simulink model "serial_spi__MAX11300"  (R2016b)
settings: Solver=FixedStepDiscrete  StartTime=0.0  StopTime=50  FixedStep=1e-3  RelTol=1e-3
undefined symbols (not defined in the file or in its folder): Ended, Single
libraries: mbed_spi_max11300 x8, mbed_lib x4
settings Model: Creator=oh  LastModifiedBy=oh
settings DataIOCC: LimitDataPoints=on  SaveFormat=Array
settings OptimizationCC: LifeSpan=1
settings DebuggingCC: SFUnexpectedBacktrackingDiag=warning  SFNoUnconditionalDefaultTransitionDiag=warning  SFExecutionAtInitializationDiag=none
settings HardwareCC: ProdBitPerPointer=32  ProdBitPerSizeT=32  ProdBitPerPtrDiffT=32  ProdLargestAtomicInteger=Long  ProdLargestAtomicFloat=Double  ProdIntDivRoundTo=Undefined  ProdWordSize=32  ProdHWDeviceType=ARM Compatible->ARM Cortex
settings ModelReferenceCC: PropagateSignalLabelsOutOfModel=off
settings RTWCC: SystemTargetFile=mbed.tlc  TemplateMakefile=mbed.tmf  Description=Mbed Target (Embedded Target)  TargetLang=C++
settings CodeAppCC: IgnoreCustomStorageClasses=off
settings STFCustomTargetCC: TargetLibSuffix=.a  GenerateSampleERTMain=on  CombineOutputUpdateFcns=on  ERTCustomFileBanners=on  SupportContinuousTime=off  SupportNonInlinedSFcns=off  RemoveResetFunc=on  MATLABClassNameForMDSCustomization=Simulink.SoftwareTarget.ERTCustomization  GRTInterface=off  SystemTargetFile=mbed.tlc
settings ERTTargetCC: GenerateSampleERTMain=on  ParMdlRefBuildCompliant=off  CompOptLevelCompliant=off  ConcurrentExecutionCompliant=off  ERTFirstTimeCompliant=off  ModelStepFunctionPrototypeControlCompliant=off  CPPClassGenCompliant=off  UseToolchainInfoCompliant=off  ERTCustomFileTemplate=mbed_file_process.tlc  ConvertIfToSwitch=off  SuppressUnreachableDefaultCases=off
settings ConfigComp: CovMetricSettings=dw  CovHtmlReporting=on  CovSaveCumulativeToWorkspaceVar=on  CovSaveSingleToWorkspaceVar=on  CovExternalEMLEnable=off

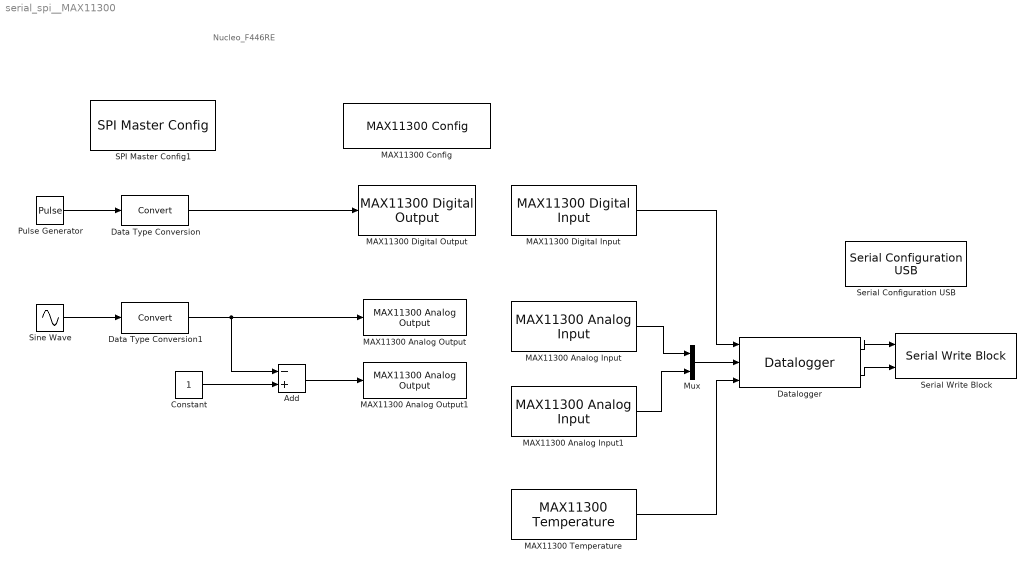
== system serial_spi__MAX11300 ==
  note: Nucleo_F446RE
  Add : Sum  Inputs=-+
  Constant : Constant  OutDataTypeStr=single
  Data Type Conversion : DataTypeConversion
  Data Type Conversion1 : DataTypeConversion
  Datalogger : mbed_lib/Utilities/Datalogger  TypeInputPorts={ 'int8' 1 'int16' 2 'single' 1 }  TypeOfInputs={'1*uint8' '2*int16' '1*single'}  BufferSize=100  errEn=off  SampleTime=0.5
  MAX11300 Analog Input : mbed_spi_max11300/MAX11300 Analog Input  CsPort=B  CsPin=6  InputType=Single-Ended  Mode=raw  PosPin=11  NegPin=0  Power=1  Range=0 to +10  Ref=Internal (2.5 V)  SampleTime=1e-3
  MAX11300 Analog Input1 : mbed_spi_max11300/MAX11300 Analog Input  CsPort=B  CsPin=6  InputType=Single-Ended  Mode=raw  PosPin=12  NegPin=0  Power=1  Range=0 to +10  Ref=Internal (2.5 V)  SampleTime=1e-3
  MAX11300 Analog Output : mbed_spi_max11300/MAX11300 Analog Output  CsPort=B  CsPin=6  Pin=1  Mode=relative  Range=0 to +10 V  SampleTime=-1
  MAX11300 Analog Output1 : mbed_spi_max11300/MAX11300 Analog Output  CsPort=B  CsPin=6  Pin=2  Mode=relative  Range=0 to +10 V  SampleTime=-1
  MAX11300 Config : mbed_spi_max11300/MAX11300 Config  Priority=1  SpiPort=1  CsPort=B  CsPin=6  AdcRate=200 kSPS  DacRef=Internal (2.5 V)  TempCh0=off  TempCh1=off  TempCh2=off
  MAX11300 Digital Input : mbed_spi_max11300/MAX11300 Digital Input  CsPort=B  CsPin=6  Pin=0  Thresh=1638  SampleTime=1e-3
  MAX11300 Digital Output : mbed_spi_max11300/MAX11300 Digital Output  CsPort=B  CsPin=6  Pin=0  Level=4095  SampleTime=-1
  MAX11300 Temperature : mbed_spi_max11300/MAX11300 Temperature  CsPort=B  CsPin=6  Channel=Internal  SampleTime=1e-3
  Mux : Mux  Inputs=2
  Pulse Generator : DiscretePulseGenerator  PulseType=Time based  Period=4  PulseWidth=50
  SPI Master Config1 : mbed_lib/Serial/SPI/SPI Master Config  Priority=0  SPIPort=1  Freq=100000  Mode=0  Bits=8  MOSIPortNameShow=A  MOSIPortName=0  MOSIPinNumber=7  MISOPortNameShow=A  MISOPortName=0  MISOPinNumber=6  SCLKPortName=A  Parameter13=0  SCLKPinNumber=5
  Serial Configuration USB : mbed_lib/Serial/UART/Serial Configuration USB  BaudRate=57600
  Serial Write Block : mbed_lib/Serial/UART/Serial Write Block  SerialPort=0  numData=on  SampleTime=-1
  Sine Wave : Sin  Amplitude=0.5  Bias=0.5  Frequency=0.05  SampleTime=1e-3
  wires:
  Pulse Generator/1 -> Data Type Conversion/1
  Data Type Conversion/1 -> MAX11300 Digital Output/1
  Sine Wave/1 -> Data Type Conversion1/1
  Add/1 -> MAX11300 Analog Output1/1
  Data Type Conversion1/1 -> Add/1, MAX11300 Analog Output/1
  MAX11300 Analog Input/1 -> Mux/1
  Datalogger/1 -> Serial Write Block/1
  Datalogger/2 -> Serial Write Block/2
  MAX11300 Analog Input1/1 -> Mux/2
  Constant/1 -> Add/2
  MAX11300 Temperature/1 -> Datalogger/3
  Mux/1 -> Datalogger/2
  MAX11300 Digital Input/1 -> Datalogger/1
